simulink model "adc_test"  (R2017b)
settings: Solver=VariableStepAuto  StartTime=0.0  StopTime=10.0  RelTol=1e-3
values from neighbouring files (symbols this model uses):
  delta = 0    [adc_gen_sim.m]
  Fs = 45158400.0    (= 45158400)    [adc_gen_sim.m]
  N = 32768    [adc_gen_sim.m]
  NCOMPARATORI = 15    [adc_gen_sim.m]
  R = 1024    [adc_gen_sim.m]
  Ts = 2.2144274376417234e-08    (= 2.21442743764e-08)    [adc_gen_sim.m]
undefined symbols (not defined in the file or in its folder): argo, clock
libraries: SDtoolbox x7
settings Model: Creator=jialinlu  LastModifiedBy=jialinlu

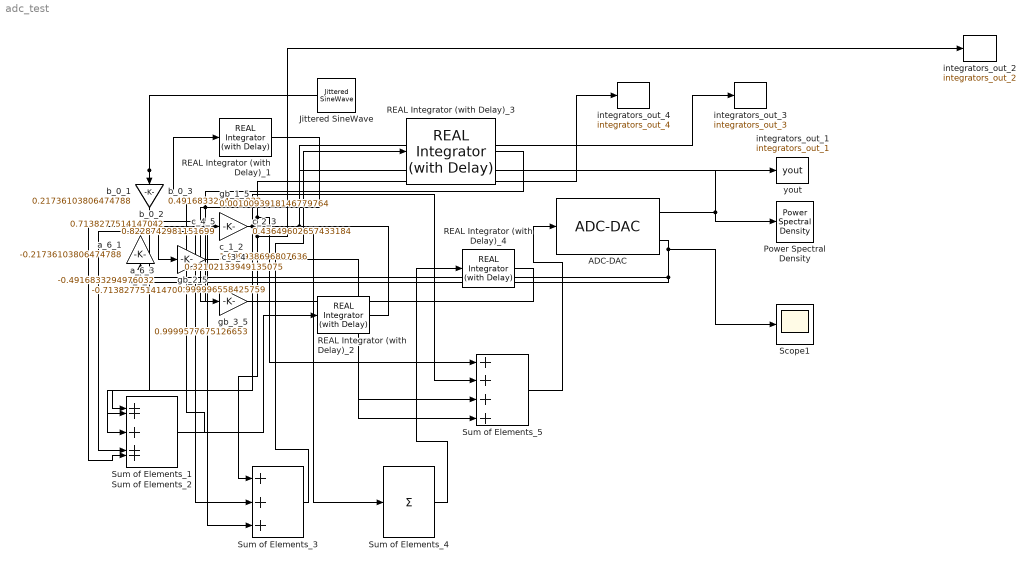
== system adc_test ==
  ADC-DAC : SDtoolbox/ADC-DAC  k=NCOMPARATORI  MM=off  match=match  CST=Cs  VVG=off  argo=argo(:,3)  LF=off  NF=retA.log
  Jittered SineWave : SDtoolbox/Jittered SineWave  Ampl=Ampl  Bias=0  Freq=finrad  Phase=0  SampJ=delta*0  Ts=Ts  seed=floor(100*sum(clock))
  Power Spectral Density : SDtoolbox/Power Spectral Density  SN=1  Fs=Fs  fBL=1  fBH=Fs/(2*R)  Fin=Fin  N=N  Ntransient=Ntransient  VW=off  savename=savemat  Scale_type=logarithmic
  REAL Integrator (with Delay)_1 : SDtoolbox/REAL Integrator (with Delay)  Ts=Ts  alfa=alfa  Amax=Amax  sr=sr  GBW=451582095.6952042
  REAL Integrator (with Delay)_2 : SDtoolbox/REAL Integrator (with Delay)  Ts=Ts  alfa=alfa  Amax=Amax  sr=sr  GBW=87809810.40111057
  REAL Integrator (with Delay)_3 : SDtoolbox/REAL Integrator (with Delay)  Ts=Ts  alfa=alfa  Amax=Amax  sr=sr  GBW=128501541.61881208
  REAL Integrator (with Delay)_4 : SDtoolbox/REAL Integrator (with Delay)  Ts=Ts  alfa=alfa  Amax=Amax  sr=sr  GBW=451583779.6181194
  Scope1 : Scope
  Sum of Elements_1 : Sum
  Sum of Elements_2 : Sum  Inputs=+++
  Sum of Elements_3 : Sum  Inputs=+++
  Sum of Elements_4 : Sum  Inputs=+
  Sum of Elements_5 : Sum  Inputs=++++
  a_6_1 : Gain  Gain=-0.21736103806474788  SaturateOnIntegerOverflow=on  OutDataTypeStr=Inherit: Same as input  ParamDataTypeStr=Inherit: Same as input
  a_6_2 : Gain  Gain=-0.7138277514147042  SaturateOnIntegerOverflow=on  OutDataTypeStr=Inherit: Same as input  ParamDataTypeStr=Inherit: Same as input
  a_6_3 : Gain  Gain=-0.4916833294976032  SaturateOnIntegerOverflow=on  OutDataTypeStr=Inherit: Same as input  ParamDataTypeStr=Inherit: Same as input
  b_0_1 : Gain  Gain=0.21736103806474788  SaturateOnIntegerOverflow=on  OutDataTypeStr=Inherit: Same as input  ParamDataTypeStr=Inherit: Same as input
  b_0_2 : Gain  Gain=0.7138277514147042  SaturateOnIntegerOverflow=on  OutDataTypeStr=Inherit: Same as input  ParamDataTypeStr=Inherit: Same as input
  b_0_3 : Gain  Gain=0.4916833294976032  SaturateOnIntegerOverflow=on  OutDataTypeStr=Inherit: Same as input  ParamDataTypeStr=Inherit: Same as input
  c_1_2 : Gain  Gain=1.999938696807636  SaturateOnIntegerOverflow=on  OutDataTypeStr=Inherit: Same as input  ParamDataTypeStr=Inherit: Same as input
  c_2_3 : Gain  Gain=0.43649602657433184  SaturateOnIntegerOverflow=on  OutDataTypeStr=Inherit: Same as input  ParamDataTypeStr=Inherit: Same as input
  c_3_4 : Gain  Gain=0.32102133949135075  SaturateOnIntegerOverflow=on  OutDataTypeStr=Inherit: Same as input  ParamDataTypeStr=Inherit: Same as input
  c_4_5 : Gain  Gain=0.8228742981151699  SaturateOnIntegerOverflow=on  OutDataTypeStr=Inherit: Same as input  ParamDataTypeStr=Inherit: Same as input
  gb_1_5 : Gain  Gain=0.0010093918146779764  SaturateOnIntegerOverflow=on  OutDataTypeStr=Inherit: Same as input  ParamDataTypeStr=Inherit: Same as input
  gb_2_5 : Gain  Gain=0.999996558425759  SaturateOnIntegerOverflow=on  OutDataTypeStr=Inherit: Same as input  ParamDataTypeStr=Inherit: Same as input
  gb_3_5 : Gain  Gain=0.9999577675126653  SaturateOnIntegerOverflow=on  OutDataTypeStr=Inherit: Same as input  ParamDataTypeStr=Inherit: Same as input
  integrators_out_1 : ToWorkspace  VariableName=integrators_out_1  SampleTime=-1
  integrators_out_2 : ToWorkspace  VariableName=integrators_out_2  SampleTime=-1
  integrators_out_3 : ToWorkspace  VariableName=integrators_out_3  SampleTime=-1
  integrators_out_4 : ToWorkspace  VariableName=integrators_out_4  SampleTime=-1
  yout : ToWorkspace  VariableName=yout  SampleTime=-1
  wires:
  ADC-DAC/1 -> Power Spectral Density/1, yout/1
  ADC-DAC/2 -> a_6_2/1, a_6_3/1, a_6_1/1, Scope1/1
  Sum of Elements_1/1 -> REAL Integrator (with Delay)_1/1
  Sum of Elements_2/1 -> REAL Integrator (with Delay)_2/1
  Sum of Elements_3/1 -> REAL Integrator (with Delay)_3/1
  Sum of Elements_4/1 -> REAL Integrator (with Delay)_4/1
  Sum of Elements_5/1 -> ADC-DAC/1
  REAL Integrator (with Delay)_1/1 -> c_1_2/1, gb_1_5/1
  c_1_2/1 -> Sum of Elements_2/1, integrators_out_1/1
  REAL Integrator (with Delay)_2/1 -> c_2_3/1, gb_2_5/1
  c_2_3/1 -> Sum of Elements_3/1, integrators_out_2/1
  REAL Integrator (with Delay)_3/1 -> c_3_4/1, gb_3_5/1
  c_3_4/1 -> Sum of Elements_4/1, integrators_out_3/1
  REAL Integrator (with Delay)_4/1 -> c_4_5/1
  c_4_5/1 -> Sum of Elements_5/1, integrators_out_4/1
  Jittered SineWave/1 -> b_0_1/1, b_0_2/1, b_0_3/1
  b_0_1/1 -> Sum of Elements_1/1
  b_0_2/1 -> Sum of Elements_2/2
  b_0_3/1 -> Sum of Elements_3/2
  a_6_1/1 -> Sum of Elements_1/2
  a_6_2/1 -> Sum of Elements_2/3
  a_6_3/1 -> Sum of Elements_3/3
  gb_1_5/1 -> Sum of Elements_5/2
  gb_2_5/1 -> Sum of Elements_5/3
  gb_3_5/1 -> Sum of Elements_5/4
